simulink model "C172S_NonlinearAutopilot_V1"  (R2026a)
settings: Solver=ode4  StartTime=0  StopTime=120  FixedStep=0.01
InitFcn:
  | na1Model=c172sNonlinearAutopilotClosedLoopData();
  | if ~strcmp(na1Model.artifactRevision,'NONLINEAR-AUTOPILOT-V1-CLOSED-LOOP-MATLAB-R1'), error('Nonlinear-autopilot closed-loop revision mismatch.'); end
  | if ~exist('na1InputSignal','var'), error('na1InputSignal is required.'); end
settings Model: Creator=Shahi  LastModifiedBy=Shahi

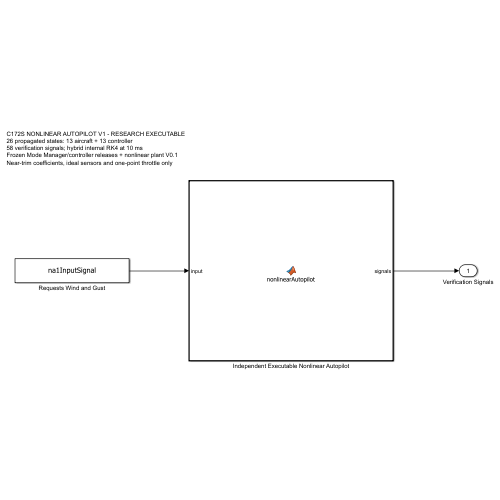
[thumbnail: Simulink's stored preview of the top-level diagram]
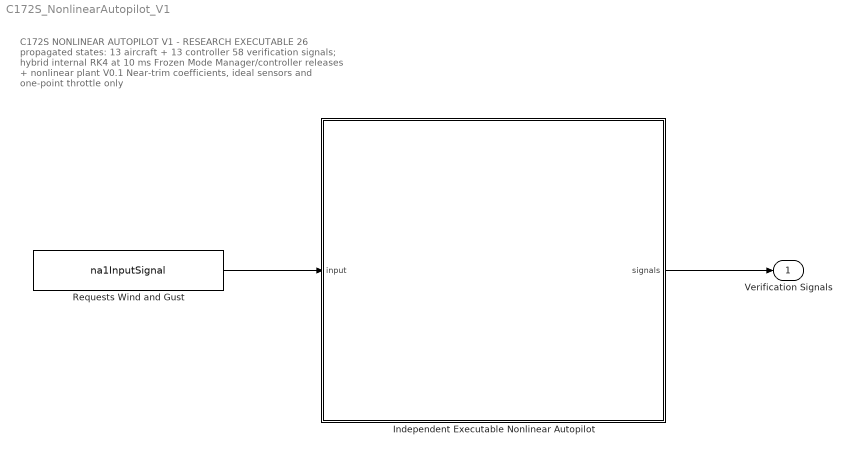
== system C172S_NonlinearAutopilot_V1 ==
  note: C172S NONLINEAR AUTOPILOT V1 - RESEARCH EXECUTABLE
      | 26 propagated states: 13 aircraft + 13 controller
      | 58 verification signals; hybrid internal RK4 at 10 ms
      | Frozen Mode Manager/controller releases + nonlinear plant V0.1
      | Near-trim coefficients, ideal sensors and one-point throttle only
  Independent Executable Nonlinear Autopilot : MATLAB Function  TreatAsAtomicUnit=on
  Requests Wind and Gust : FromWorkspace  VariableName=na1InputSignal  SampleTime=0.01  Interpolate=off  OutputAfterFinalValue=Holding final value
  Verification Signals : Outport
  wires:
  Requests Wind and Gust/1 -> Independent Executable Nonlinear Autopilot/1(input)
  Independent Executable Nonlinear Autopilot/1(signals) -> Verification Signals/1

== matlab function C172S_NonlinearAutopilot_V1/Independent Executable Nonlinear Autopilot ==
  settings: updateMethod=DISCRETE  sampleTime=0.01
  data: input input; signals output
function signals = nonlinearAutopilot(input)
%#codegen
persistent initialized z managerInitialized engaged lateralMode verticalMode
persistent bankRef pitchRef headingRef altitudeRef coreTimer headingTimer altitudeTimer
persistent aileronTimer elevatorTimer delayR delayP delayPhi delayPsi
persistent previousAileronSaturated previousElevatorSaturated
if isempty(initialized)
z=[56.588888888888846;0;-1.8576028133659581e-16;0;0;0;0;0;-1219.2;1;0;-1.6413140899561787e-18;0;zeros(13,1)];
managerInitialized=false; engaged=false; lateralMode=uint8(0); verticalMode=uint8(0);
bankRef=0.0; pitchRef=0.0; headingRef=0.0; altitudeRef=4000.0;
coreTimer=0.0; headingTimer=0.0; altitudeTimer=0.0; aileronTimer=0.0; elevatorTimer=0.0;
delayR=0.0; delayP=0.0; delayPhi=0.0; delayPsi=zeros(5,1);
previousAileronSaturated=false; previousElevatorSaturated=false; initialized=true;
end
request=input(1:19); wind=input(20:22); gust=input(23:25);
[phi0,theta0,psi0,qNorm0]=attitude(z(10:13));
altitudeFt0=-z(9)/0.3048;
coreValid0=all(isfinite(z(4:6))) && isfinite(qNorm0) && abs(qNorm0-1.0)<=1.0e-8;
headingValid0=coreValid0 && isfinite(psi0); altitudeValid0=isfinite(altitudeFt0);
if ~managerInitialized
bankRef=captureBank(phi0*180/pi); pitchRef=clip(theta0*180/pi,-3.0,3.0);
headingRef=normalizeHeading(psi0*180/pi); altitudeRef=altitudeFt0;
delayR=z(6); delayP=z(4); delayPhi=phi0; delayPsi(:)=psi0; managerInitialized=true;
end
[engaged,lateralMode,verticalMode,bankRef,pitchRef,headingRef,altitudeRef,...
 coreTimer,headingTimer,altitudeTimer,aileronTimer,elevatorTimer,...
 rollTrack,pitchTrack,eventCode]=managerStep(engaged,lateralMode,verticalMode,...
 bankRef,pitchRef,headingRef,altitudeRef,coreTimer,headingTimer,altitudeTimer,...
 aileronTimer,elevatorTimer,request,phi0,theta0,coreValid0,...
 headingValid0,altitudeValid0,previousAileronSaturated,previousElevatorSaturated);
headingEnable=engaged && lateralMode==uint8(2); altitudeEnable=engaged && verticalMode==uint8(2);
bankCommand=0.0; pitchCommand=0.0;
if engaged && lateralMode==uint8(1), bankCommand=bankRef; end
if engaged && verticalMode==uint8(1), pitchCommand=pitchRef; end
if pitchTrack
z(14)=theta0; pitchError=z(14)-theta0;
z(15)=(-0.45000000000000001*pitchError+0.12*z(5)-z(16))/0.45000000000000001;
end
if rollTrack
z(25)=phi0; bankError=z(25)-z(22);
z(23)=(z(24)-0.29999999999999999*bankError+0.074999999999999997*z(21))/0.089999999999999997;
end
supervisor=[double(engaged);double(headingEnable);double(altitudeEnable);bankCommand;
 pitchCommand;headingRef;altitudeRef];
delays=[delayR;delayP;delayPhi;delayPsi(1)];
[k1,diagnostic]=closedRhs(z,supervisor,delays,wind,gust);
signals=[z;diagnostic(1:18);double(engaged);double(lateralMode);double(verticalMode);
 double(rollTrack);double(pitchTrack);double(eventCode);bankCommand;pitchCommand;
 headingRef;altitudeRef;diagnostic(19);diagnostic(20);aileronTimer;elevatorTimer];
previousAileronSaturated=diagnostic(19)~=0;
previousElevatorSaturated=diagnostic(20)~=0;
sampleR=z(6); sampleP=z(4); samplePhi=phi0; samplePsi=psi0;
k2=closedRhs(z+0.005*k1,supervisor,delays,wind,gust);
k3=closedRhs(z+0.005*k2,supervisor,delays,wind,gust);
k4=closedRhs(z+0.01*k3,supervisor,delays,wind,gust);
z=z+(0.01/6.0)*(k1+2.0*k2+2.0*k3+k4);
z(10:13)=z(10:13)/sqrt(sum(z(10:13).^2));
delayR=sampleR; delayP=sampleP; delayPhi=samplePhi; delayPsi=[delayPsi(2:5);samplePsi];
end

function [engaged,lateralMode,verticalMode,bankRef,pitchRef,headingRef,altitudeRef,...
 coreTimer,headingTimer,altitudeTimer,aileronTimer,elevatorTimer,...
 rollTrack,pitchTrack,eventCode]=managerStep(engaged,lateralMode,verticalMode,...
 bankRef,pitchRef,headingRef,altitudeRef,coreTimer,headingTimer,altitudeTimer,...
 aileronTimer,elevatorTimer,r,phi,theta,coreValid,headingValid,...
 altitudeValid,previousASat,previousESat)
dt=0.01; rollTrack=false; pitchTrack=false; eventCode=uint8(0); wasEngaged=engaged;
inputCore=(r(5)~=0)&&coreValid; inputHeading=(r(6)~=0)&&headingValid;
inputAltitude=(r(7)~=0)&&altitudeValid; inputASat=(r(8)~=0)||previousASat;
inputESat=(r(9)~=0)||previousESat;
coreTimer=timerUpdate(~inputCore,coreTimer,dt);
headingTimer=timerUpdate(~inputHeading,headingTimer,dt);
altitudeTimer=timerUpdate(~inputAltitude,altitudeTimer,dt);
aileronTimer=timerUpdate(inputASat,aileronTimer,dt);
elevatorTimer=timerUpdate(inputESat,elevatorTimer,dt);
if engaged
if r(2)~=0, engaged=false; eventCode=uint8(7);
elseif r(3)~=0, engaged=false; eventCode=uint8(8);
elseif abs(phi*180/pi)>30.0 || abs(theta*180/pi)>10.0, engaged=false; eventCode=uint8(11);
elseif coreTimer+eps>=0.10, engaged=false; eventCode=uint8(9);
elseif max(aileronTimer,elevatorTimer)+eps>=2.0, engaged=false; eventCode=uint8(10);
end
if ~engaged, lateralMode=uint8(0); verticalMode=uint8(0); end
end
if ~engaged
if ~wasEngaged && r(1)~=0
permitted=(r(4)~=0)&&inputCore&&(r(3)==0)&&~inputASat&&~inputESat;
if r(10)==2, permitted=permitted&&inputHeading; end
if r(11)==2, permitted=permitted&&inputAltitude; end
if permitted
engaged=true; eventCode=uint8(1); rollTrack=true; pitchTrack=true;
if r(10)==2, lateralMode=uint8(2); headingRef=normalizeHeading(r(18));
else, lateralMode=uint8(1); bankRef=captureBank(phi*180/pi); end
if r(11)==2, verticalMode=uint8(2); altitudeRef=r(19);
else, verticalMode=uint8(1); pitchRef=clip(theta*180/pi,-3.0,3.0); end
else, eventCode=uint8(4);
end
end
return
end
if lateralMode==uint8(2) && headingTimer+eps>=0.10
lateralMode=uint8(1); bankRef=captureBank(phi*180/pi); rollTrack=true; eventCode=uint8(5);
end
if verticalMode==uint8(2) && altitudeTimer+eps>=0.10
verticalMode=uint8(1); pitchRef=clip(theta*180/pi,-3.0,3.0); pitchTrack=true; eventCode=uint8(6);
end
if r(10)~=0
if r(10)==1, lateralMode=uint8(1); bankRef=captureBank(phi*180/pi); rollTrack=true; eventCode=uint8(2);
elseif r(10)==2 && inputHeading, lateralMode=uint8(2); headingRef=normalizeHeading(r(18)); rollTrack=true; eventCode=uint8(2);
else, eventCode=uint8(3); end
end
if r(11)~=0
if r(11)==1, verticalMode=uint8(1); pitchRef=clip(theta*180/pi,-3.0,3.0); pitchTrack=true; eventCode=uint8(2);
elseif r(11)==2 && inputAltitude, verticalMode=uint8(2); altitudeRef=r(19); pitchTrack=true; eventCode=uint8(2);
else, eventCode=uint8(3); end
end
if lateralMode==uint8(2) && r(12)~=0 && inputHeading, headingRef=normalizeHeading(r(18)); end
if verticalMode==uint8(2) && r(13)~=0 && inputAltitude, altitudeRef=r(19); end
end

function [zDot,d]=closedRhs(z,sup,delay,wind,gust)
control=[z(16);z(24);z(20);0.65];
[xDot,TAS,alpha,beta]=plantRhs(z(1:13),control,wind,gust);
[phi,theta,psi,qNorm]=attitude(z(10:13)); altitudeFt=-z(9)/0.3048;
altitudePerturbation=-z(9)-1219.2; verticalSpeed=-xDot(9);
altitudeCommand=(sup(7)-4000.0)*0.3048;
verticalCommand=clip(0.59999999999999998*(z(17)-altitudePerturbation),-1.5240000000000031,1.5240000000000031);
thetaOuter=clip(0.02*(verticalCommand-verticalSpeed),-0.05235987755982989,0.05235987755982989);
if sup(3)~=0, thetaSelected=thetaOuter; else, thetaSelected=sup(5)*pi/180; end
pitchError=z(14)-theta;
eUnsat=-0.45000000000000001*pitchError-0.45000000000000001*z(15)+0.12*z(5);
eLimited=clip(eUnsat,-0.087266462599716474,0.087266462599716474);
eTarget=sup(1)*eLimited;
eRateRaw=(eTarget-z(16))/0.035000000000000003;
eRate=clip(eRateRaw,-0.3490658503988659,0.3490658503988659);
eTrack=z(16)+0.035000000000000003*eRate;
pitchAW=(eUnsat-eTrack)/(0.45000000000000001*0.5);
headingError=wrapAngle(sup(6)*pi/180-z(26));
bankOuter=clip(0.57499999999999996*headingError,-0.3490658503988659,0.3490658503988659);
if sup(2)~=0, bankSelected=bankOuter; else, bankSelected=sup(4)*pi/180; end
yawWash=z(18)-z(19);
rUnsat=-0.28000000000000003*yawWash;
rLimited=clip(rUnsat,-0.087266462599716474,0.087266462599716474);
rTarget=sup(1)*rLimited;
rRateRaw=(rTarget-z(20))/0.050000000000000003;
rRate=clip(rRateRaw,-0.3490658503988659,0.3490658503988659);
bankError=z(25)-z(22);
aUnsat=0.29999999999999999*bankError+0.089999999999999997*z(23)-0.074999999999999997*z(21);
aLimited=clip(aUnsat,-0.087266462599716474,0.087266462599716474);
aTarget=sup(1)*aLimited;
aRateRaw=(aTarget-z(24))/0.050000000000000003;
aRate=clip(aRateRaw,-0.52359877559829882,0.52359877559829882);
aTrack=z(24)+0.050000000000000003*aRate;
rollAW=(aTrack-aUnsat)/(0.089999999999999997*0.5);
cDot=zeros(13,1);
cDot(1)=(thetaSelected-z(14))/2;
cDot(2)=pitchError+pitchAW; cDot(3)=eRate;
cDot(4)=(altitudeCommand-z(17))/5;
cDot(5)=(delay(1)-z(18))/0.02;
cDot(6)=(z(18)-z(19))/1;
cDot(7)=rRate;
cDot(8)=(delay(2)-z(21))/0.02;
cDot(9)=(delay(3)-z(22))/0.02;
cDot(10)=bankError+rollAW; cDot(11)=aRate;
cDot(12)=(bankSelected-z(25))/2;
cDot(13)=(delay(4)-z(26))/0.10000000000000001;
zDot=[xDot;cDot];
tol=1.0e-12; eSat=(sup(1)~=0)&&((abs(eUnsat-eLimited)>tol)||(abs(eRateRaw-eRate)>tol));
aSat=(sup(1)~=0)&&((abs(aUnsat-aLimited)>tol)||(abs(aRateRaw-aRate)>tol));
within=(TAS>=80*0.514444444444444)&&(TAS<=130*0.514444444444444)&&...
 (alpha>=-4*pi/180)&&(alpha<=10*pi/180)&&(beta>=-8*pi/180)&&(beta<=8*pi/180)&&...
 (phi>=-30*pi/180)&&(phi<=30*pi/180)&&(theta>=-10*pi/180)&&(theta<=10*pi/180);
d=[control;eRate;aRate;rRate;phi;theta;psi;altitudeFt;altitudePerturbation;
 verticalSpeed;TAS;alpha;beta;qNorm;double(within);double(aSat);double(eSat)];
end

function [xdot,TAS,alpha,beta]=plantRhs(x,u,steadyWind,gust)
wind=steadyWind+gust;
[f0,~,~,~,~,~,airVelocity,windBody]=evaluatePlant(x,u,wind,0.0);
[f1,~,~,~,~,~,~,~]=evaluatePlant(x,u,wind,1.0);
omega=x(4:6); a0=f0(1:3)+cross(omega,windBody); a1=f1(1:3)+cross(omega,windBody);
r0=alphaRate(airVelocity,a0); r1=alphaRate(airVelocity,a1); alphaDot=r0/(1.0-(r1-r0));
[xdot,TAS,alpha,beta,~,~,~,~]=evaluatePlant(x,u,wind,alphaDot);
end

function rate=alphaRate(v,a)
rate=(v(1)*a(3)-v(3)*a(1))/(v(1)^2+v(3)^2);
end

function [xdot,TAS,alpha,beta,F,M,airVelocity,windBody]=evaluatePlant(x,u,wind,alphaDot)
mass=1156.6605434999999; gravity=9.8066499999999994;
I=[1424.9552348898205 0 -0;0 1828.6803192734997 0;-0 0 2956.6740184607975];
q=x(10:13); q=q/sqrt(sum(q.^2)); q0=q(1);q1=q(2);q2=q(3);q3=q(4);
C=[q0^2+q1^2-q2^2-q3^2,2*(q1*q2-q0*q3),2*(q1*q3+q0*q2);
 2*(q1*q2+q0*q3),q0^2-q1^2+q2^2-q3^2,2*(q2*q3-q0*q1);
 2*(q1*q3-q0*q2),2*(q2*q3+q0*q1),q0^2-q1^2-q2^2+q3^2];
windBody=C'*wind; airVelocity=x(1:3)-windBody; TAS=sqrt(sum(airVelocity.^2));
alpha=atan2(airVelocity(3),airVelocity(1)); beta=asin(min(1,max(-1,airVelocity(2)/TAS)));
temperature=288.14999999999998-0.0064999999999999997*(-x(9));
pressure=101325*(temperature/288.14999999999998)^(9.8066499999999994/(287.05286999999998*0.0064999999999999997));
rho=pressure/(287.05286999999998*temperature);
qbarS=0.5*rho*TAS^2*16.165128960000001;
pHat=x(4)*10.91184/(2*TAS);qHat=x(5)*1.49352/(2*TAS);rHat=x(6)*10.91184/(2*TAS);
adHat=alphaDot*1.49352/(2*TAS);
CL=0.40283185525292292+5.5*alpha+3.8799999999999999*qHat+1.49*adHat+0.42699999999999999*u(1);
CD=0.035628731280772659+0.25*alpha;
CY=-0.31*beta+-0.036999999999999998*pHat+0.20999999999999999*rHat+-0*u(2)+-0.187*u(3);
Cl=-0.088999999999999996*beta+-0.46999999999999997*pHat+0.096000000000000002*rHat+0.17799999999999999*u(2)+-0.0147*u(3);
Cm=-0.93794217687074832*alpha+-11.4*qHat+-4.3600000000000003*adHat+-1.26*u(1);
Cn=0.065000000000000002*beta+-0.029999999999999999*pHat+-0.099000000000000005*rHat+0.052999999999999999*u(2)+0.065699999999999995*u(3);
L=qbarS*CL;D=qbarS*CD;Y=qbarS*CY;thrust=u(4)*1543.4401413548464;
Fa=[-D*cos(alpha)+L*sin(alpha);Y;-D*sin(alpha)-L*cos(alpha)];
F=Fa+thrust*[cos(alpha);0;sin(alpha)];
M=[qbarS*10.91184*Cl;qbarS*1.49352*Cm;qbarS*10.91184*Cn];
omega=x(4:6);gravityBody=C'*[0;0;gravity];
vdot=F/mass+gravityBody-cross(omega,x(1:3));
H=I*omega;odot=I\(M-cross(omega,H));pdot=C*x(1:3);
qv=q(2:4);Q=[-qv';q0*eye(3)+[0 -qv(3) qv(2);qv(3) 0 -qv(1);-qv(2) qv(1) 0]];
qdot=0.5*Q*omega;xdot=[vdot;odot;pdot;qdot];
end

function [phi,theta,psi,qNorm]=attitude(q)
qNorm=sqrt(sum(q.^2));q=q/qNorm;q0=q(1);q1=q(2);q2=q(3);q3=q(4);
phi=atan2(2*(q0*q1+q2*q3),1-2*(q1^2+q2^2));
argument=min(1,max(-1,2*(q0*q2-q3*q1)));theta=asin(argument);
psi=atan2(2*(q0*q3+q1*q2),1-2*(q2^2+q3^2));psi=mod(psi,2*pi);
end

function value=timerUpdate(condition,previous,dt)
if condition,value=previous+dt;else,value=0.0;end
end
function value=captureBank(bank)
if abs(bank)<6.0,value=0.0;else,value=clip(bank,-20.0,20.0);end
end
function value=normalizeHeading(value)
value=mod(value,360.0);if value<0.0,value=value+360.0;end
end
function value=wrapAngle(value)
value=mod(value+pi,2*pi)-pi;
end
function value=clip(value,lower,upper)
value=min(max(value,lower),upper);
end
